simulink model "Model_kyvadla_na_voziku_m_slx"  (R2020a)
settings: Solver=FixedStepAuto  StartTime=0.0  StopTime=50  FixedStep=0.01  RelTol=1e-3
values from neighbouring files (symbols this model uses):
  g = 9.81    [run_wout_simmech.m]
  m = 15    [run_wout_simmech.m]
  M = 5    [run_wout_simmech.m]
undefined symbols (not defined in the file or in its folder): f, l
settings Model: Creator=Jiří  LastModifiedBy=Jiří

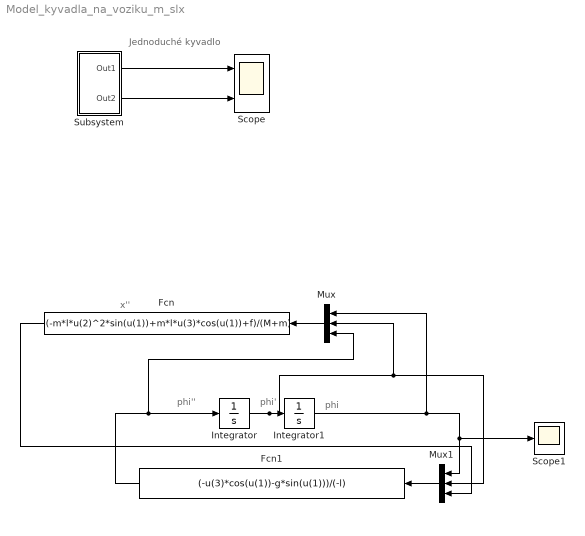
== system Model_kyvadla_na_voziku_m_slx ==
  note: phi
  note: phi'
  note: phi''
  note: x''
  note: Jednoduché kyvadlo
  Fcn : Fcn  Expr=(-m*l*u(2)^2*sin(u(1))+m*l*u(3)*cos(u(1))+f)/(M+m)
  Fcn1 : Fcn  Expr=(-u(3)*cos(u(1))-g*sin(u(1)))/(-l)
  Integrator : Integrator
  Integrator1 : Integrator  InitialCondition=2
  Mux : Mux  Inputs=3
  Mux1 : Mux  Inputs=3
  Scope : Scope  NumInputPorts=2
  Scope1 : Scope
  Subsystem : Subsystem
  wires:
  Subsystem/1(Out1) -> Scope/1
  Subsystem/2(Out2) -> Scope/2
  Mux/1 -> Fcn/1
  Fcn/1 -> Mux1/3
  Integrator/1 -> Mux/2, Mux1/2, Integrator1/1
  Fcn1/1 -> Mux/3, Integrator/1
  Mux1/1 -> Fcn1/1
  Integrator1/1 -> Mux/1, Scope1/1, Mux1/1

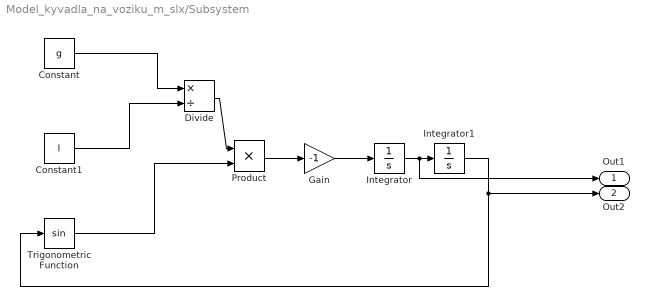
== system Model_kyvadla_na_voziku_m_slx/Subsystem ==
  Constant : Constant  Value=g
  Constant1 : Constant  Value=l
  Divide : Product  Inputs=*/
  Gain : Gain  Gain=-1
  Integrator : Integrator
  Integrator1 : Integrator  InitialCondition=1
  Product : Product
  Trigonometric Function : Trigonometry
  Out1 : Outport
  Out2 : Outport  Port=2
  wires:
  Gain/1 -> Integrator/1
  Integrator/1 -> Out1/1, Integrator1/1
  Constant/1 -> Divide/1
  Trigonometric Function/1 -> Product/2
  Divide/1 -> Product/1
  Product/1 -> Gain/1
  Constant1/1 -> Divide/2
  Integrator1/1 -> Out2/1, Trigonometric Function/1
